simulink model "TrafficLightROS"  (R2022b)
settings: Solver=VariableStepAuto  StartTime=0.0  StopTime=10.0  RelTol=1e-3
undefined symbols (not defined in the file): Data, Data_SL_Info
libraries: MainLibrary x9, robotlib x1
settings Model: Creator=20211327  LastModifiedBy=20211327

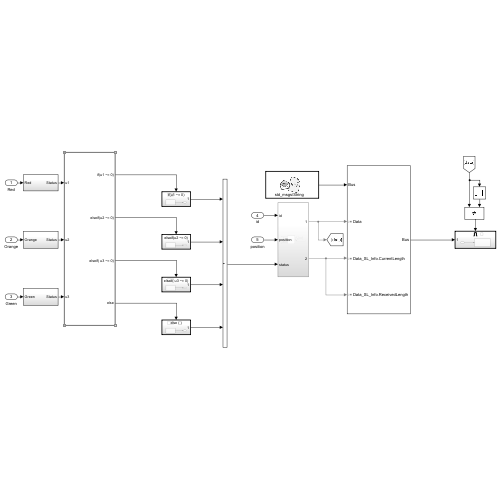
[thumbnail: Simulink's stored preview of the top-level diagram]
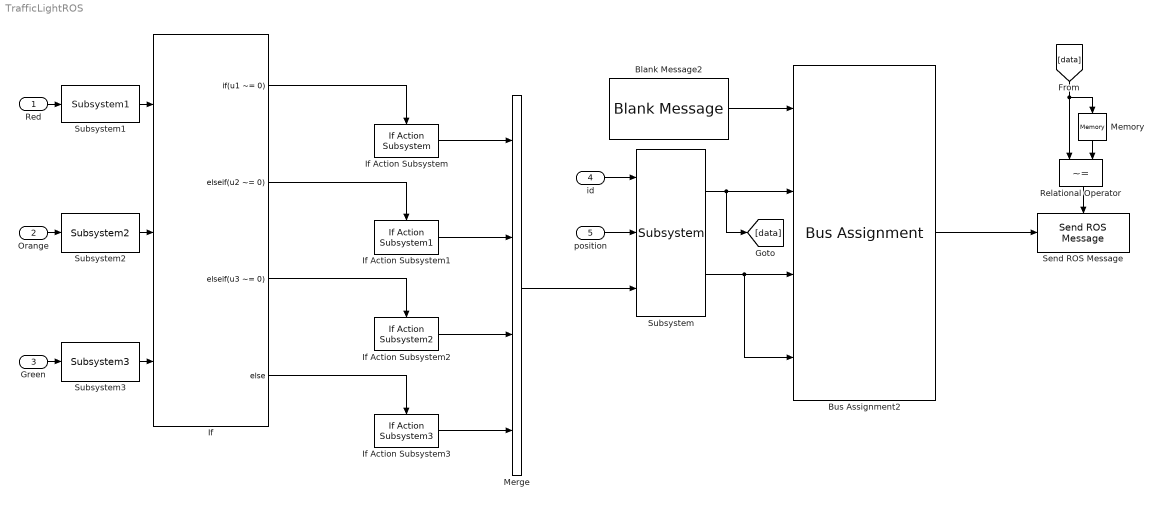
== system TrafficLightROS ==
  Red : Inport
  Orange : Inport  Port=2
  Green : Inport  Port=3
  id : Inport  Port=4
  position : Inport  Port=5
  Blank Message2 : robotlib/Blank Message  messageClass=Message  entityType=std_msgs/String  messageType=std_msgs/String  SampleTime=inf  legacyBusStruct=off
  Bus Assignment2 : BusAssignment  AssignedSignals=Data,Data_SL_Info.CurrentLength,Data_SL_Info.ReceivedLength
  If : If  NumInputs=3  IfExpression=u1 ~= 0  ElseIfExpressions=u2 ~= 0, u3 ~= 0
  If Action Subsystem : MainLibrary/TrafficLight2ROSmessage/Traffic Light Ros Message/If Action Subsystem  SystemSampleTime=-1  VariantActivationTime=update diagram  Latency=0  AutoFrameSizeCalculation=off
      settings: SourceProductName=Custom_Prescan-ROS_Library
  If Action Subsystem1 : MainLibrary/TrafficLight2ROSmessage/Traffic Light Ros Message/If Action Subsystem1  SystemSampleTime=-1  VariantActivationTime=update diagram  Latency=0  AutoFrameSizeCalculation=off
      settings: SourceProductName=Custom_Prescan-ROS_Library
  If Action Subsystem2 : MainLibrary/TrafficLight2ROSmessage/Traffic Light Ros Message/If Action Subsystem2  SystemSampleTime=-1  VariantActivationTime=update diagram  Latency=0  AutoFrameSizeCalculation=off
      settings: SourceProductName=Custom_Prescan-ROS_Library
  If Action Subsystem3 : MainLibrary/TrafficLight2ROSmessage/Traffic Light Ros Message/If Action Subsystem3  SystemSampleTime=-1  VariantActivationTime=update diagram  Latency=0  AutoFrameSizeCalculation=off
      settings: SourceProductName=Custom_Prescan-ROS_Library
  Memory : Memory  InitialCondition=zeros(1,128)
  Merge : Merge  Inputs=4
  Relational Operator : RelationalOperator  Operator=~=  OutDataTypeStr=boolean  RndMeth=Simplest  InputSameDT=off
  Send ROS Message : MainLibrary/TrafficLight2ROSmessage/Traffic Light Ros Message/Send ROS Message  SystemSampleTime=-1  VariantActivationTime=update diagram  Latency=0  AutoFrameSizeCalculation=off
      settings: SourceProductName=Custom_Prescan-ROS_Library
  Subsystem : MainLibrary/TrafficLight2ROSmessage/Traffic Light Ros Message/Subsystem  SystemSampleTime=-1  VariantActivationTime=update diagram  Latency=0  AutoFrameSizeCalculation=off
      settings: SourceProductName=Custom_Prescan-ROS_Library
  Subsystem1 : MainLibrary/TrafficLight2ROSmessage/Traffic Light Ros Message/Subsystem1  SystemSampleTime=-1  VariantActivationTime=update diagram  Latency=0  AutoFrameSizeCalculation=off
      settings: SourceProductName=Custom_Prescan-ROS_Library
  Subsystem2 : MainLibrary/TrafficLight2ROSmessage/Traffic Light Ros Message/Subsystem2  SystemSampleTime=-1  VariantActivationTime=update diagram  Latency=0  AutoFrameSizeCalculation=off
      settings: SourceProductName=Custom_Prescan-ROS_Library
  Subsystem3 : MainLibrary/TrafficLight2ROSmessage/Traffic Light Ros Message/Subsystem3  SystemSampleTime=-1  VariantActivationTime=update diagram  Latency=0  AutoFrameSizeCalculation=off
      settings: SourceProductName=Custom_Prescan-ROS_Library
  wires:
  Subsystem2/1 -> If/2
  Red/1 -> Subsystem1/1
  Subsystem/2 -> Bus Assignment2/4, Bus Assignment2/3
  If Action Subsystem/1 -> Merge/1
  If/1 -> If Action Subsystem/Action
  If/4 -> If Action Subsystem3/Action
  If Action Subsystem2/1 -> Merge/3
  Bus Assignment2/1 -> Send ROS Message/1
  id/1 -> Subsystem/1
  position/1 -> Subsystem/2
  If/2 -> If Action Subsystem1/Action
  [data] -> Relational Operator/1, Memory/1
  If Action Subsystem3/1 -> Merge/4
  Green/1 -> Subsystem3/1
  If Action Subsystem1/1 -> Merge/2
  Relational Operator/1 -> Send ROS Message/Enable
  If/3 -> If Action Subsystem2/Action
  Memory/1 -> Relational Operator/2
  Merge/1 -> Subsystem/3
  Subsystem1/1 -> If/1
  Subsystem3/1 -> If/3
  Orange/1 -> Subsystem2/1
  Blank Message2/1 -> Bus Assignment2/1
  Subsystem/1 -> [data], Bus Assignment2/2
